simulink model "SP_CV2S"  (R2025b)
settings: Solver=VariableStepAuto  StartTime=0.0  StopTime=500  RelTol=1e-6
values from neighbouring files (symbols this model uses):
  g = 9.81    [SP_CV2.m]
  h_0 = 1    [SP_CV2.m]
  h_max = 2    [SP_CV2.m]
  k = 1/c    [SP_CV2.m]
  mu = 0.62    [SP_CV2.m]
  q10 = mu * S0 * sqrt(2 * g * h_0)    [SP_CV2.m]
  q20 = q10    [SP_CV2.m]
  S = 1    [SP_CV2.m]
  S0 = 0.01    [SP_CV2.m]
  T = S/c    [SP_CV2.m]
settings Model: Creator=jakub  LastModifiedBy=jakub

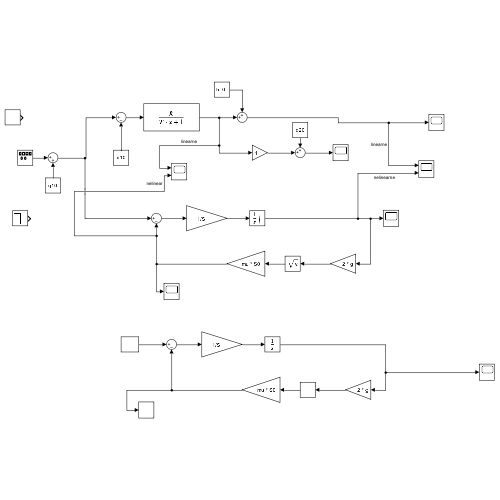
[thumbnail: Simulink's stored preview of the top-level diagram]
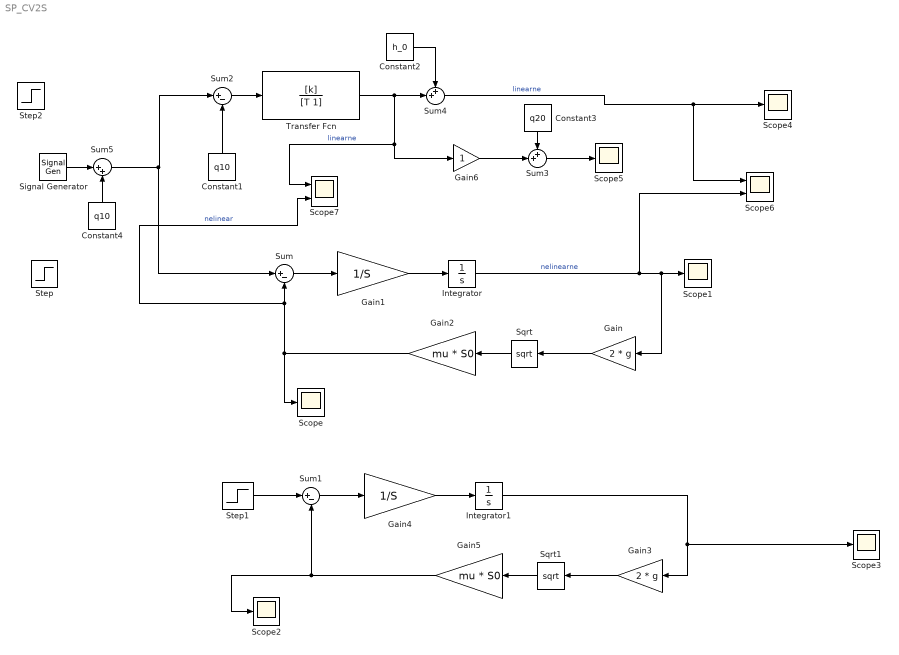
== system SP_CV2S ==
  Constant1 : Constant  Value=q10
  Constant2 : Constant  Value=h_0
  Constant3 : Constant  Value=q20
  Constant4 : Constant  Value=q10
  Gain : Gain  Gain=2 * g
  Gain1 : Gain  Gain=1/S
  Gain2 : Gain  Gain=mu * S0
  Gain3 : Gain  Gain=2 * g
  Gain4 : Gain  Gain=1/S
  Gain5 : Gain  Gain=mu * S0
  Gain6 : Gain
  Integrator : Integrator  InitialCondition=1  LimitOutput=on  UpperSaturationLimit=h_max  LowerSaturationLimit=0
  Integrator1 : Integrator
  Scope{,1..5} (6 alike) : Scope
      Scope settings: ActiveDisplayYMinimum=-0.0050556906084998094  ActiveDisplayYMaximum=0.016018854700153219
      Scope1 settings: ActiveDisplayYMinimum=-0.32760461358028509  ActiveDisplayYMaximum=0.98489538641971508
      Scope2 settings: ActiveDisplayYMinimum=-0.0050556906084998094  ActiveDisplayYMaximum=0.016018854700153219  DataLoggingVariableName=ScopeData2
      Scope3 settings: ActiveDisplayYMinimum=-0.12499999999999997  ActiveDisplayYMaximum=1.125  DataLoggingVariableName=ScopeData3
      Scope4 settings: ActiveDisplayYMinimum=-144.41393808607157  ActiveDisplayYMaximum=338.50233234755126  DataLoggingVariableName=ScopeData4
      Scope5 settings: ActiveDisplayYMinimum=-57.87182260466264  ActiveDisplayYMaximum=285.32775480858186  DataLoggingVariableName=ScopeData5
  Scope6 : Scope  NumInputPorts=2
      settings: ActiveDisplayYMinimum=-0.52363723972699627  ActiveDisplayYMaximum=2.148479864490394  DataLoggingVariableName=ScopeData6
  Scope7 : Scope  NumInputPorts=2
      settings: ActiveDisplayYMinimum=-2404.2990337377828  ActiveDisplayYMaximum=610.01167411835991  DataLoggingVariableName=ScopeData7
  Signal Generator : SignalGenerator  WaveForm=square  Amplitude=0.005  Frequency=0.1571  Units=rad/sec
  Sqrt : Sqrt
  Sqrt1 : Sqrt
  Step : Step  Before=q10  After=0  SampleTime=0
  Step1 : Step  After=q10  SampleTime=0
  Step2 : Step  Before=q10  After=0  SampleTime=0
  Sum : Sum  Inputs=|+-
  Sum1 : Sum  Inputs=|+-
  Sum2 : Sum  Inputs=|+-
  Sum3 : Sum  Inputs=++|
  Sum4 : Sum  Inputs=++|
  Sum5 : Sum  Inputs=|++
  Transfer Fcn : TransferFcn  Numerator=[k]  Denominator=[T 1]
  wires:
  Gain/1 -> Sqrt/1
  Sqrt/1 -> Gain2/1
  Gain2/1 -> Scope/1, Scope7/2, Sum/2  "nelinear"
  Sum/1 -> Gain1/1
  Gain1/1 -> Integrator/1
  Integrator/1 -> Scope6/2, Scope1/1, Gain/1  "nelinearne"
  Gain4/1 -> Integrator1/1
  Integrator1/1 -> Scope3/1, Gain3/1
  Gain3/1 -> Sqrt1/1
  Sqrt1/1 -> Gain5/1
  Gain5/1 -> Scope2/1, Sum1/2
  Step1/1 -> Sum1/1
  Sum1/1 -> Gain4/1
  Sum2/1 -> Transfer Fcn/1
  Transfer Fcn/1 -> Scope7/1, Gain6/1, Sum4/2  "linearne"
  Constant1/1 -> Sum2/2
  Constant2/1 -> Sum4/1
  Gain6/1 -> Sum3/2
  Constant3/1 -> Sum3/1
  Sum4/1 -> Scope6/1, Scope4/1  "linearne"
  Sum3/1 -> Scope5/1
  Signal Generator/1 -> Sum5/1
  Sum5/1 -> Sum/1, Sum2/1
  Constant4/1 -> Sum5/2
